simulink model "s17042023_6a"  (R2021b)
settings: Solver=VariableStepAuto  StartTime=0  StopTime=0.1  RelTol=1e-3
libraries: spsSeriesRLCBranchLib x10, spsVoltageMeasurementLib x4, spsACVoltageSourceLib x3, spsUniversalBridgeLib x2, spsCurrentMeasurementLib x1, spsGroundLib x1, spsPWMGenerator2LevelLib x1, spspowerguiLib x1, spsSeriesRLCLoadLib x1
settings Model: PacingRate=4  Creator=Иванов  LastModifiedBy=79159
settings SolverCC: ZeroCrossAlgorithm=Adaptive
settings DataIOCC: SaveFormat=StructureWithTime  ReturnWorkspaceOutputs=off
settings DebuggingCC: IgnoredZcDiagnostic=none

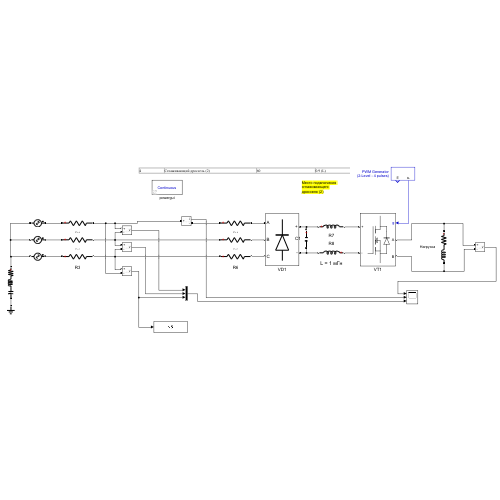
[thumbnail: Simulink's stored preview of the top-level diagram]
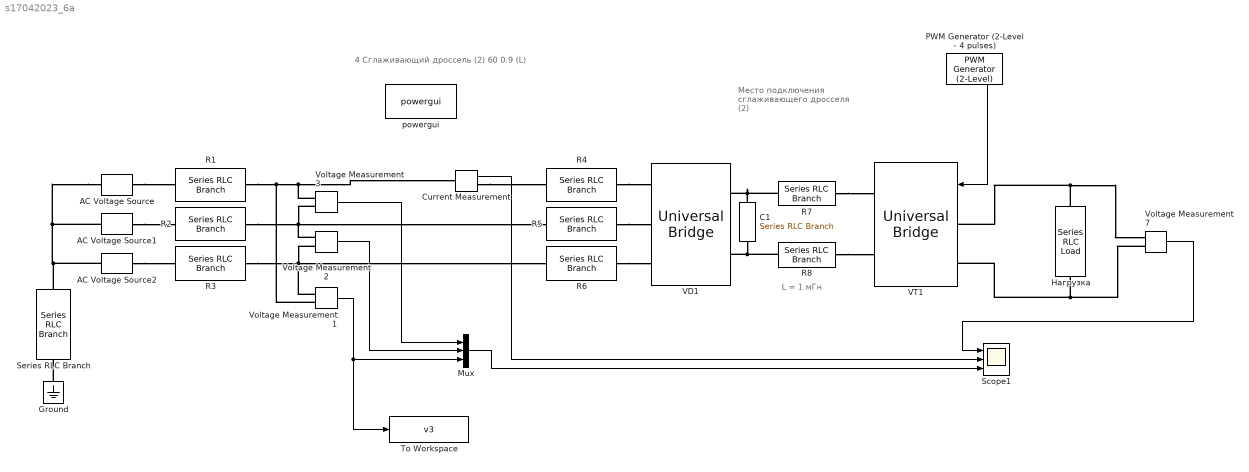
== system s17042023_6a ==
  note: 4
      | Сглаживающий дроссель (2)
      | 60
      | 0.9 (L)
  note: Место подключения
      | сглаживающего
      | дросселя (2)
  note: L = 1 мГн
  AC Voltage Source : spsACVoltageSourceLib/AC Voltage Source  Amplitude=220*sqrt(2)  Phase=0  Frequency=50  SampleTime=0  Measurements=None  BusType=swing  Pref=10e3  Qref=0  Qmin=-inf  Qmax=+inf
  AC Voltage Source1 : spsACVoltageSourceLib/AC Voltage Source  Amplitude=220*sqrt(2)  Phase=120  Frequency=50  SampleTime=0  Measurements=None  BusType=swing  Pref=10e3  Qref=0  Qmin=-inf  Qmax=+inf
  AC Voltage Source2 : spsACVoltageSourceLib/AC Voltage Source  Amplitude=220*sqrt(2)  Phase=-120  Frequency=50  SampleTime=0  Measurements=None  BusType=swing  Pref=10e3  Qref=0  Qmin=-inf  Qmax=+inf
  C1 : spsSeriesRLCBranchLib/Series RLC Branch  LConnTagsString=__new0  RConnTagsString=__new0  BranchType=C  Resistance=0  Inductance=0  SetiL0=off  InitialCurrent=0  Capacitance=8800e-6  Setx0=on  InitialVoltage=0  Measurements=None
  Current Measurement : spsCurrentMeasurementLib/Current Measurement  PhasorSimulation=off  OutputType=Complex  PSBequivalent=0
  Ground : spsGroundLib/Ground  LConnTagsString=a
  Mux : Mux  Inputs=3
  PWM Generator (2-Level - 4 pulses) : spsPWMGenerator2LevelLib/PWM Generator (2-Level)  ModulatorType=Single-phase full-bridge (4 pulses)  ModulatorMode=Unsynchronized  Fc=60000  Pc=0  nF=27  MinMax="[ -1  1 ]"  SamplingTechnique=Natural  ModulatingSignals=on  m=0.8  Freq=66000  Phase=0  Ts=4e-6  ShowCarrierOutport=on
  R1 : spsSeriesRLCBranchLib/Series RLC Branch  LConnTagsString=__new0  RConnTagsString=__new0  BranchType=R  Resistance=0.4  Inductance=0  SetiL0=off  InitialCurrent=0  Capacitance=38e-6  Setx0=off  InitialVoltage=0  Measurements=None
  R{2,4..6} (4 alike) : spsSeriesRLCBranchLib/Series RLC Branch  LConnTagsString=__new0  RConnTagsString=__new0  BranchType=R  Resistance=0.4  Inductance=0  SetiL0=off  InitialCurrent=0  Capacitance=0  Setx0=off  InitialVoltage=0  Measurements=None
  R3 : spsSeriesRLCBranchLib/Series RLC Branch  LConnTagsString=__new0  RConnTagsString=__new0  BranchType=R  Resistance=0.4  Inductance=0  SetiL0=off  InitialCurrent=0  Capacitance=38e-6  Setx0=off  InitialVoltage=0  Measurements=None
  R7 : spsSeriesRLCBranchLib/Series RLC Branch  LConnTagsString=__new0  RConnTagsString=__new0  BranchType=L  Resistance=0.4  Inductance=1e-3  SetiL0=off  InitialCurrent=0.05  Capacitance=0  Setx0=off  InitialVoltage=0  Measurements=None
  R8 : spsSeriesRLCBranchLib/Series RLC Branch  LConnTagsString=__new0  RConnTagsString=__new0  BranchType=L  Resistance=0.4  Inductance=1e-3  SetiL0=off  InitialCurrent=0.05  Capacitance=0  Setx0=off  InitialVoltage=0  Measurements=None
  Scope1 : Scope  NumInputPorts=3
  Series RLC Branch : spsSeriesRLCBranchLib/Series RLC Branch  LConnTagsString=__new0  RConnTagsString=__new0  BranchType=RLC  Resistance=4  Inductance=0  SetiL0=off  InitialCurrent=0  Capacitance=0  Setx0=off  InitialVoltage=0  Measurements=None
  To Workspace : ToWorkspace  VariableName=v3  SaveFormat=Structure With Time  SampleTime=-1
  VD1 : spsUniversalBridgeLib/Universal Bridge  Arms=3  SnubberResistance=1e5  SnubberCapacitance=10e-12  Device=Diodes  Ron=1e-3  Lon=0  ForwardVoltages="[  0  0  ]"  ForwardVoltage=0.5  GTOparameters=[ 10e-6 , 20e-6 ]  IGBTparameters=[ 1e-6 , 2e-6 ]  Measurements=Device voltages  Measurements_2=None  converterType=Rectifier
  VT1 : spsUniversalBridgeLib/Universal Bridge  Arms=2  SnubberResistance=1e5  SnubberCapacitance=200e-12  Device=MOSFET / Diodes  Ron=0.2e-3  Lon=0  ForwardVoltages="[  0  0  ]"  ForwardVoltage=0  GTOparameters=[ 10e-6 , 20e-6 ]  IGBTparameters=[ 1e-6 , 2e-6 ]  Measurements=None  Measurements_2=None  converterType=Rectifier
  Voltage Measurement{1..3,7} (4 alike) : spsVoltageMeasurementLib/Voltage Measurement  PhasorSimulation=off  OutputType=Complex  PSBequivalent=0
  powergui : spspowerguiLib/powergui  Priority=1  SimulationMode=Continuous  SampleTime=2e-6  frequency=60  Iterations=50  frequencyindice=50  Pbase=100e6  ErrMax=1e-4  UnitsV=kV  UnitsW=MW  buscounter=0  FunctionMessages=off  echomessages=off  EnableUseOfTLC=off  CurrentSourceSwitches=off  DisableSnubberDevices=off  DisableRonSwitches=off  DisableVfSwitches=off  DisplayEquations=off  AutomaticDiscreteSolvers=off  SolverType=Tustin/Backward Euler (TBE)  Interpol=off  ExternalGateDelay=off  methode=off  Ts=100  x0status=blocks  SPID=on  SwTol=0  HookPort=off  NonlinearTolerance=1e-4  nMaxIteration=100  ContinueOnMaxIteration=off  RestoreLinks=warning  ResistiveCurrentMeasurement=off  Frange=[0:2:500]  Ylog=off  Xlog=on  ShowGrid=off  save=off  variable=ZData  structure=0  ZoomFFT=off  StartTime=0.0  cycles=1  DisplayStyle=1  fundamental=60  FreqAxis=off  MaxFrequency=1000  frequencyindicesteady=1  RmsSteady=1  display=off
  Нагрузка : spsSeriesRLCLoadLib/Series RLC Load  LConnTagsString=a  RConnTagsString=__new0  NominalVoltage=380  NominalFrequency=66000  ActivePower=60000  InductivePower=29059  CapacitivePower=0  Setx0=off  InitialVoltage=0  SetiL0=off  InitialCurrent=0  Measurements=None  LoadType=constant Z
  wires:
  PWM Generator (2-Level - 4 pulses)/1 -> VT1/1
  Voltage Measurement3/1 -> Mux/1
  Voltage Measurement2/1 -> Mux/2
  Voltage Measurement1/1 -> Mux/3, To Workspace/1
  Mux/1 -> Scope1/3
  Current Measurement/1 -> Scope1/2
  Voltage Measurement7/1 -> Scope1/1
  connections:
  Ground/LConn1 -- Series RLC Branch/RConn1
  VT1/LConn1 -- Нагрузка/LConn1 -- Voltage Measurement7/LConn1
  Voltage Measurement7/LConn2 -- Нагрузка/RConn1 -- VT1/LConn2
  AC Voltage Source/RConn1 -- R1/LConn1
  AC Voltage Source1/RConn1 -- R2/LConn1
  R4/RConn1 -- VD1/LConn1
  R5/RConn1 -- VD1/LConn2
  R6/RConn1 -- VD1/LConn3
  AC Voltage Source/LConn1 -- Series RLC Branch/LConn1 -- AC Voltage Source2/LConn1 -- AC Voltage Source1/LConn1
  AC Voltage Source2/RConn1 -- R3/LConn1
  Current Measurement/RConn1 -- R4/LConn1
  R1/RConn1 -- Voltage Measurement1/LConn2 -- Voltage Measurement3/LConn1 -- Current Measurement/LConn1
  R2/RConn1 -- Voltage Measurement3/LConn2 -- Voltage Measurement2/LConn1 -- R5/LConn1
  R3/RConn1 -- Voltage Measurement2/LConn2 -- Voltage Measurement1/LConn1 -- R6/LConn1
  R7/LConn1 -- C1/LConn1 -- VD1/RConn1
  C1/RConn1 -- VD1/RConn2 -- R8/RConn1
  R8/LConn1 -- VT1/RConn2
  R7/RConn1 -- VT1/RConn1
